simulink model "ShiftArithemetic_model"  (R2016b)
settings: Solver=VariableStepAuto  StartTime=0.0  StopTime=10.0  RelTol=1e-3
values from neighbouring files (symbols this model uses):
  byte0_int32 = int32(bin2dec(byte0_bit_pattern))    [TEST_ShiftArithmetic.m]
  byte1_int32 = int32(bin2dec(byte1_bit_pattern))    [TEST_ShiftArithmetic.m]
  byte2_int32 = int32(bin2dec(byte2_bit_pattern))    [TEST_ShiftArithmetic.m]
  byte3_int32 = int32(bin2dec(byte3_bit_pattern))    [TEST_ShiftArithmetic.m]
settings Model: Creator=Christopher  LastModifiedBy=Christopher

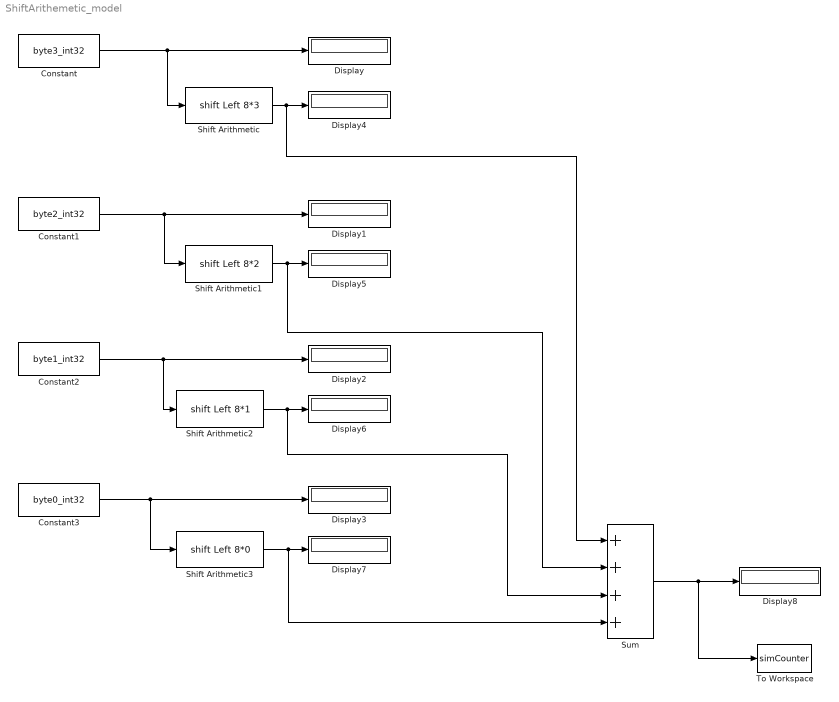
== system ShiftArithemetic_model ==
  Constant : Constant  Value=byte3_int32
  Constant1 : Constant  Value=byte2_int32
  Constant2 : Constant  Value=byte1_int32
  Constant3 : Constant  Value=byte0_int32
  Display{,1..8} (9 alike) : Display
  Shift Arithmetic : ArithShift  BitShiftNumber=8*3  BitShiftDirection=Left
  Shift Arithmetic1 : ArithShift  BitShiftNumber=8*2  BitShiftDirection=Left
  Shift Arithmetic2 : ArithShift  BitShiftNumber=8*1  BitShiftDirection=Left
  Shift Arithmetic3 : ArithShift  BitShiftNumber=8*0  BitShiftDirection=Left
  Sum : Sum  Inputs=++++
  To Workspace : ToWorkspace  VariableName=simCounter  SaveFormat=Structure With Time  SampleTime=-1
  wires:
  Constant/1 -> Shift Arithmetic/1, Display/1
  Constant1/1 -> Shift Arithmetic1/1, Display1/1
  Constant2/1 -> Shift Arithmetic2/1, Display2/1
  Constant3/1 -> Shift Arithmetic3/1, Display3/1
  Shift Arithmetic/1 -> Sum/1, Display4/1
  Shift Arithmetic1/1 -> Sum/2, Display5/1
  Shift Arithmetic2/1 -> Sum/3, Display6/1
  Shift Arithmetic3/1 -> Sum/4, Display7/1
  Sum/1 -> To Workspace/1, Display8/1
